simulink model "Helicopter_linear"  (R2018a)
settings: Solver=VariableStepAuto  StartTime=0.0  StopTime=inf  RelTol=1e-3
values from neighbouring files (symbols this model uses):
  A = [A1;A2;A3;A4]    [Helicopter_Values.m]
  B = [B1;B2;B3;B4]    [Helicopter_Values.m]
  Vmp_op = (kyy*mheli*g*cos(p_r_op)*lcm)/(kyy*kpp -kyp*kpy)    [Helicopter_Values.m]
  Vmy_op = kyp*Vmp_op/kyy    [Helicopter_Values.m]
libraries: realtime_pacer_lib x1
settings Model: Creator=pacoa  LastModifiedBy=pacoa

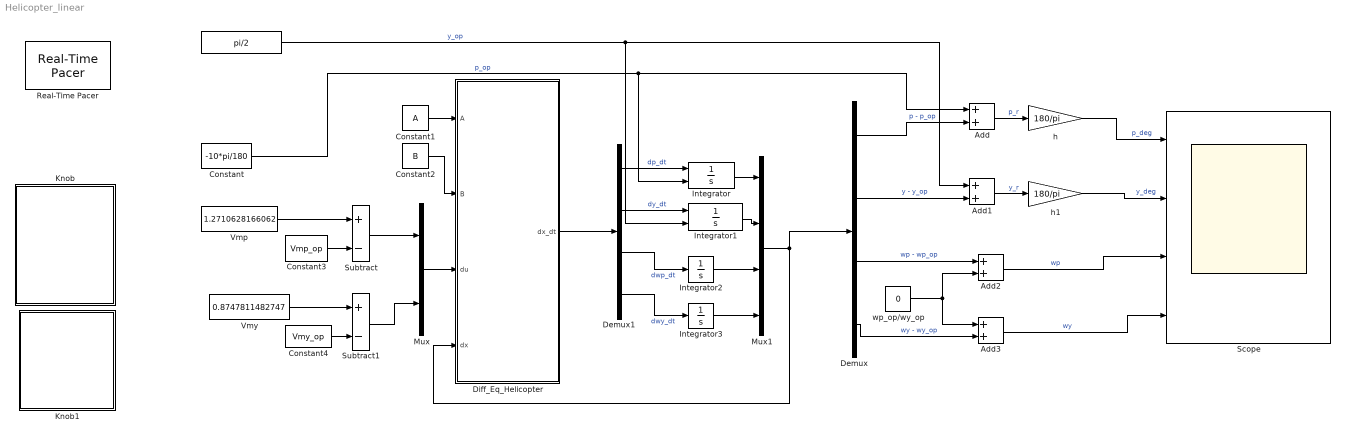
== system Helicopter_linear ==
  " " : Constant  Value=pi/2
  Add{,1..3} (4 alike) : Sum
  Constant : Constant  Value=-10*pi/180
  Constant1 : Constant  Value=A
  Constant2 : Constant  Value=B
  Constant3 : Constant  Value=Vmp_op
  Constant4 : Constant  Value=Vmy_op
  Demux : Demux
  Demux1 : Demux
  Diff_Eq_Helicopter : MATLAB Function  TreatAsAtomicUnit=on
  Integrator : Integrator  InitialConditionSource=external  InitialCondition=-10*pi/180  LimitOutput=on  UpperSaturationLimit=pi/4 - (-10*pi/180)  LowerSaturationLimit=-pi/4 - (-10*pi/180)
  Integrator1 : Integrator  InitialConditionSource=external  InitialCondition=pi/2  LimitOutput=on  UpperSaturationLimit=pi - (pi/2)  LowerSaturationLimit=0 - (pi/2)
  Integrator2 : Integrator  UpperSaturationLimit=pi
  Integrator3 : Integrator
  Knob : Subsystem  DialogController=hmiCreateDDGDialog  IsWebBlock=on  mask(MWDashboardBlock){webBlockId=2947dbe9-c983-48e5-a0e7-08dc830ec4db, webBlockType=continuousknob, ShowInLibBrowser=on, ShowInitialText=on, HMISrcModelName=Helicopter_linear}
      mask prompts: webBlockId "WebBlock Id"; webBlockType "WebBlock Type"; HMISrcModelName "Source Model"
      mask help: SimulinkHMI:dialogs:ContinuousKnobDialogDesc
      mask Help: helpview([docroot '/mapfiles/simulink.map'], 'hmi_knob')
      mask Display:
      | if strcmp(get_param(bdroot(gcb),'BlockDiagramType'), 'library')
      |     image([(matlabroot) '/toolbox/simulink/hmi/icons/ContinuousKnob.png']);
      | end
  Knob1 : Subsystem  DialogController=hmiCreateDDGDialog  IsWebBlock=on  mask(MWDashboardBlock){webBlockId=831ebf9a-2240-453b-9ad7-4d7eab751952, webBlockType=continuousknob, ShowInLibBrowser=on, ShowInitialText=on, HMISrcModelName=Helicopter_linear}
      mask prompts: webBlockId "WebBlock Id"; webBlockType "WebBlock Type"; HMISrcModelName "Source Model"
      mask help: SimulinkHMI:dialogs:ContinuousKnobDialogDesc
      mask Help: helpview([docroot '/mapfiles/simulink.map'], 'hmi_knob')
      mask Display:
      | if strcmp(get_param(bdroot(gcb),'BlockDiagramType'), 'library')
      |     image([(matlabroot) '/toolbox/simulink/hmi/icons/ContinuousKnob.png']);
      | end
  Mux : Mux  Inputs=2
  Mux1 : Mux
  Real-Time Pacer : realtime_pacer_lib/Real-Time Pacer  simTimePerRealTime=10
  Scope : Scope  NumInputPorts=4
  Subtract : Sum  Inputs=+-
  Subtract1 : Sum  Inputs=+-
  Vmp : Constant  Value=1.2710628166062
  Vmy : Constant  Value=0.8747811482747
  h : Gain  Gain=180/pi
  h1 : Gain  Gain=180/pi
  wp_op/wy_op : Constant  Value=0
  wires:
  h1/1 -> Scope/2  "y_deg"
  h/1 -> Scope/1  "p_deg"
  " "/1 -> Add1/1, Integrator1/2  "y_op"
  Subtract/1 -> Mux/1
  Subtract1/1 -> Mux/2
  Mux/1 -> Diff_Eq_Helicopter/3(du)
  Constant/1 -> Integrator/2, Add/1  "p_op"
  Constant1/1 -> Diff_Eq_Helicopter/1(A)
  Constant2/1 -> Diff_Eq_Helicopter/2(B)
  Demux/1 -> Add/2  "p - p_op"
  Add/1 -> h/1  "p_r"
  Demux/2 -> Add1/2  "y - y_op"
  wp_op/wy_op/1 -> Add2/2, Add3/1
  Demux/4 -> Add3/2  "wy - wy_op"
  Demux/3 -> Add2/1  "wp - wp_op"
  Add1/1 -> h1/1  "y_r"
  Add2/1 -> Scope/3  "wp"
  Add3/1 -> Scope/4  "wy"
  Diff_Eq_Helicopter/1(dx_dt) -> Demux1/1
  Demux1/1 -> Integrator/1  "dp_dt"
  Demux1/2 -> Integrator1/1  "dy_dt"
  Demux1/3 -> Integrator2/1  "dwp_dt"
  Demux1/4 -> Integrator3/1  "dwy_dt"
  Integrator3/1 -> Mux1/4
  Integrator2/1 -> Mux1/3
  Integrator1/1 -> Mux1/2
  Integrator/1 -> Mux1/1
  Mux1/1 -> Demux/1, Diff_Eq_Helicopter/4(dx)
  Vmp/1 -> Subtract/1
  Constant4/1 -> Subtract1/2
  Vmy/1 -> Subtract1/1
  Constant3/1 -> Subtract/2

== system Helicopter_linear/Knob ==

== system Helicopter_linear/Knob1 ==

== matlab function Helicopter_linear/Diff_Eq_Helicopter ==
  data: A input; B input; du input size=[2 1]; dx_dt output; dx input size=[4 1]
function dx_dt = fcn(A,B,du,dx)

dx_dt =A*dx + B*(du);
